simulink model "lab5"  (R2017b)
settings: Solver=VariableStepAuto  StartTime=0.0  StopTime=10.0  RelTol=1e-3
InitFcn:
  | load speech_signal;
  | Fs = 8000;
  | Ts = 1/Fs;
  | 
  | Data_size = 2048;
  | Address_size = 12;
  | Upscale = 32;
undefined symbols (not defined in the file): Radix
libraries: hdlsllib x9, simulink x5, dspmtrx3 x4, dspxfrm3 x2, dspsigops x2, dspvision x1, dspsnks4 x1
settings Model: Creator=Ross_admin  LastModifiedBy=s15z586
settings OptimizationCC: BlockReduction=off  ConditionallyExecuteInputs=off  DefaultParameterBehavior=Inlined
settings DebuggingCC: AlgebraicLoopMsg=error
settings HardwareCC: ProdBitPerPointer=32  ProdBitPerSizeT=32  ProdBitPerPtrDiffT=32  ProdLargestAtomicFloat=None  ProdIntDivRoundTo=Undefined  ProdEndianess=Unspecified  ProdWordSize=32  ProdHWDeviceType=ASIC/FPGA->ASIC/FPGA  TargetBitPerPointer=64  TargetBitPerSizeT=64  TargetBitPerPtrDiffT=64  TargetLongLongMode=on  TargetIntDivRoundTo=Zero  TargetEndianess=LittleEndian  TargetWordSize=64  TargetHWDeviceType=Custom Processor->MATLAB Host Computer  ProdEqTarget=off
settings CodeAppCC: StateflowObjectComments=on

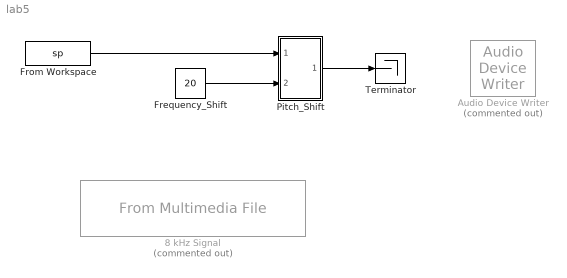
== system lab5 ==
  8 kHz Signal : dspvision/From Multimedia File  Commented=on  inputFilename=SpeechDFT-16-8-mono-5secs.wav  loop=on  numPlays=1  outputStreams=Audio only  videoDataType=single  audioDataType=double  inheritSampleTime=on  userDefinedSampleTime=1/30  noAudioOutput=off  isIntensityVideo=off  fourcc=RGB  colorVideoFormat=Separate color signals  outputEOF=off  dataOrg=Column-major  audioFrameSize=1024  computeAudioFrameSize=off  outSamplingMode=Sample based
      settings: SourceProductBaseCode=VP
  Audio Device Writer : dspsnks4/Audio Device Writer  Commented=on  Driver=DirectSound  Device=Default  InheritSampleRate=on  SampleRate=44100  BitDepth=16-bit integer  BufferSize=4096  NumBuffers=10  DefaultOutputChannelMapping=on  OutputChannelMapping=1:2  OutputNumUnderrunSamples=off  DriverIdx=1  DeviceWarnFlag=''
  Frequency_Shift : Constant  Value=20  OutDataTypeStr=int16
  From Workspace : FromWorkspace  VariableName=sp  SampleTime=Ts
  Pitch_Shift : Subsystem
  Terminator : Terminator
  wires:
  Frequency_Shift/1 -> Pitch_Shift/2(In2)
  From Workspace/1 -> Pitch_Shift/1(In1)
  Pitch_Shift/1(Out1) -> Terminator/1

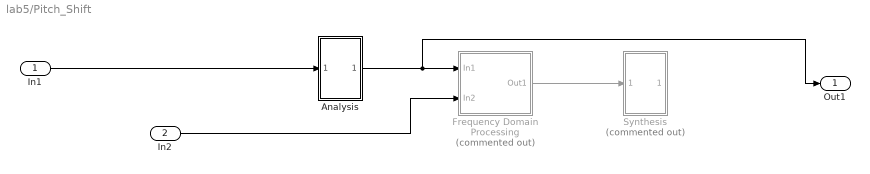
== system lab5/Pitch_Shift ==
  In1 : Inport
  In2 : Inport  Port=2
  Analysis : Subsystem
  Frequency Domain Processing : Subsystem  Commented=on
  Synthesis : Subsystem  Commented=on
  Out1 : Outport
  wires:
  In1/1 -> Analysis/1(In1)
  Frequency Domain Processing/1(Out1) -> Synthesis/1(In1)
  In2/1 -> Frequency Domain Processing/2(In2)
  Analysis/1(Out1) -> Out1/1, Frequency Domain Processing/1(In1)

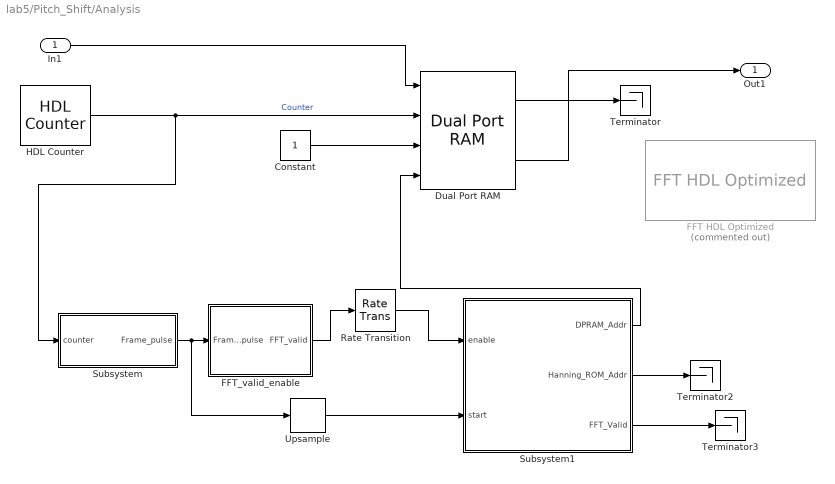
== system lab5/Pitch_Shift/Analysis ==
  In1 : Inport
  Constant : Constant  OutDataTypeStr=boolean  SampleTime=-1
  Dual Port RAM : hdlsllib/HDL RAMs/Dual Port RAM  ram_size=Address_size
      settings: SourceProductName=HDL Coder  SourceProductBaseCode=HD
  FFT HDL Optimized : dspxfrm3/FFT HDL Optimized  Commented=on  FFTLength=1024  Architecture=Burst Radix 2  ComplexMultiplication=Use 3 multipliers and 5 adders  BitReversedOutput=on  BitReversedInput=off  Normalize=off  SimulateUsing=Code generation  RoundingMethod=Floor  ResetInputPort=off  StartOutputPort=off  EndOutputPort=off
      settings: SourceProductName=DSP System Toolbox  SourceProductBaseCode=DS
  FFT_valid_enable : Subsystem
  HDL Counter : hdlsllib/Sources/HDL Counter  CountType=Count limited  CountInit=0  CountStep=1  CountMax=Data_size  CountFromType=Initial value  CountFrom=0  CountResetPort=off  CountLoadPort=off  CountEnbPort=off  CountDirPort=off  CountDataType=Unsigned  CountWordLen=12  CountFracLen=0  CountSampTime=Ts
      settings: SourceProductBaseCode=HD
  Rate Transition : RateTransition  OutPortSampleTime=Ts
  Subsystem : Subsystem
  Subsystem1 : Subsystem
  Terminator : Terminator
  Terminator2 : Terminator
  Terminator3 : Terminator
  Upsample : dspsigops/Upsample  N=4  phase=0  RateOptions=Allow multirate processing  ic=0  mode=Unused parameter value
  Out1 : Outport
  wires:
  In1/1 -> Dual Port RAM/1
  Constant/1 -> Dual Port RAM/3
  HDL Counter/1 -> Subsystem/1("counter "), Dual Port RAM/2  "Counter"
  Subsystem/1(Frame_pulse) -> Upsample/1, FFT_valid_enable/1(Frame_pulse)
  Subsystem1/1(DPRAM_Addr) -> Dual Port RAM/4
  Dual Port RAM/1 -> Terminator/1
  FFT_valid_enable/1(FFT_valid) -> Rate Transition/1
  Subsystem1/2(Hanning_ROM_Addr) -> Terminator2/1
  Subsystem1/3(FFT_Valid) -> Terminator3/1
  Dual Port RAM/2 -> Out1/1
  Rate Transition/1 -> Subsystem1/1(enable)
  Upsample/1 -> Subsystem1/2(start)

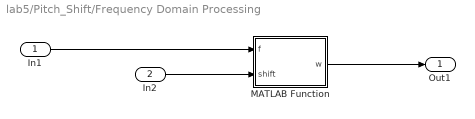
== system lab5/Pitch_Shift/Frequency Domain Processing ==
  In1 : Inport
  In2 : Inport  Port=2
  MATLAB Function : MATLAB Function  TreatAsAtomicUnit=on
  Out1 : Outport
  wires:
  In1/1 -> MATLAB Function/1(f)
  In2/1 -> MATLAB Function/2(shift)
  MATLAB Function/1(w) -> Out1/1

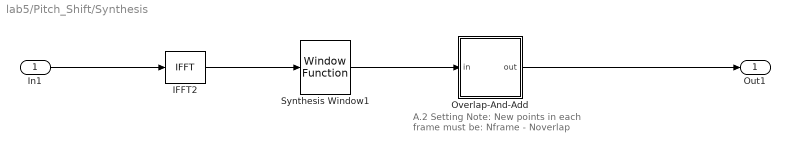
== system lab5/Pitch_Shift/Synthesis ==
  note: A.2
      | Setting Note:
      | New points in each frame must be:
      | Nframe - Noverlap
  In1 : Inport
  IFFT2 : dspxfrm3/IFFT  FFTImplementation=Radix-2  CompMethod=Table lookup  TableOpt=HYBRID  TableOptActive=Speed  BitRevOrder=off  cs_in=on  Normalize=on  InheritFFTLength=on  FFTLength=64  WrapInput=on  mode=Complex  outSamplingMode=Sample based  roundingMode=Floor  overflowMode=off  firstCoeffMode=User-defined  firstCoeffWordLength=16  firstCoeffFracLength=15  firstCoeffDataTypeStr=fixdt(1,16)  firstCoeffLastDataTypeStr=fixdt(1,16)  accumDataTypeStr=Inherit: Same as product output  accumLastDataTypeStr=Inherit: Same as product output  outputMin=[]  outputMax=[]
      settings: SourceProductName=DSP System Toolbox
  Overlap-And-Add : Subsystem  mask(Overlap-And-Add){L=1024 * 1/4}
      mask prompts: L "Number of new points in each frame"
      mask help: Performs overlap-and-add on the input signal. Disjoint frames of the input signal are overlapped with each other for a specified number of points and summed.
      mask Display: disp('Overlap\nAnd\nAdd')
  Synthesis Window1 : dspsigops/Window Function  winmode=Apply window to input  wintype=Hanning  sampmode=Continuous  samptime=1  N=64  Rs=50  beta=10  winsamp=Periodic  UserWindow=hamming  OptParams=off  UserParams={1.0}  dataType=double  isSigned=on  wordLen=16  udDataType=sfix(16)  fracBitsMode=Best precision  numFracBits=15  roundingMode=Floor  overflowMode=off  numSidelobes=4  sidelobeLevel=-30
      settings: SourceProductName=DSP System Toolbox  SourceProductBaseCode=DS
  Out1 : Outport
  wires:
  IFFT2/1 -> Synthesis Window1/1
  Synthesis Window1/1 -> Overlap-And-Add/1(in)
  Overlap-And-Add/1(out) -> Out1/1
  In1/1 -> IFFT2/1

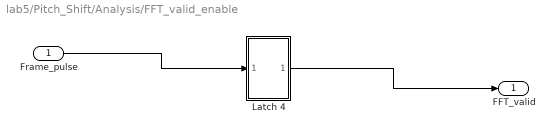
== system lab5/Pitch_Shift/Analysis/FFT_valid_enable ==
  Frame_pulse : Inport
  "Latch 4 " : Subsystem
  FFT_valid : Outport
  wires:
  Frame_pulse/1 -> "Latch 4 "/1(In1)
  "Latch 4 "/1(Out1) -> FFT_valid/1

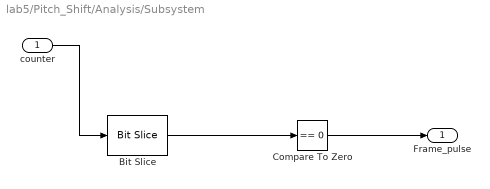
== system lab5/Pitch_Shift/Analysis/Subsystem ==
  "counter " : Inport
  Bit Slice : hdlsllib/Logic and Bit Operations/Bit Slice  lidx=7  ridx=0
  Compare To Zero : simulink/Logic and Bit Operations/Compare To Zero  relop===  OutDataTypeStr=boolean
  Frame_pulse : Outport
  wires:
  "counter "/1 -> Bit Slice/1
  Bit Slice/1 -> Compare To Zero/1
  Compare To Zero/1 -> Frame_pulse/1

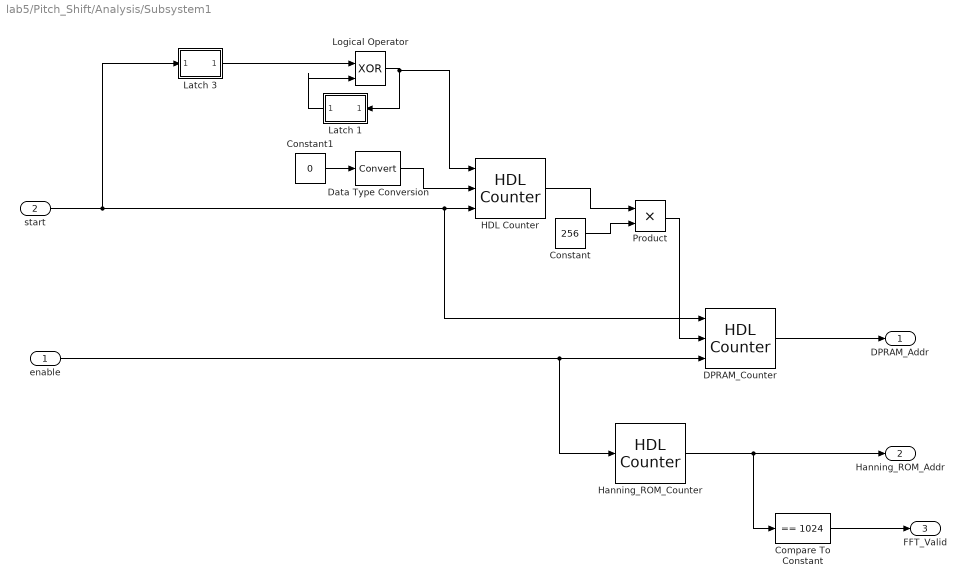
== system lab5/Pitch_Shift/Analysis/Subsystem1 ==
  enable : Inport
  start : Inport  Port=2
  Compare To Constant : simulink/Logic and Bit Operations/Compare To Constant  relop===  const=1024  OutDataTypeStr=boolean
  Constant : Constant  Value=256
  Constant1 : Constant  Value=0
  DPRAM_Counter : hdlsllib/Sources/HDL Counter  CountType=Count limited  CountInit=0  CountStep=1  CountMax=Data_size  CountFromType=Specify  CountFrom=0  CountResetPort=off  CountLoadPort=on  CountEnbPort=on  CountDirPort=off  CountDataType=Unsigned  CountWordLen=12  CountFracLen=0  CountSampTime=1
      settings: SourceProductBaseCode=HD
  Data Type Conversion : DataTypeConversion
  HDL Counter : hdlsllib/Sources/HDL Counter  CountType=Count limited  CountInit=0  CountStep=1  CountMax=1792/256  CountFromType=Initial value  CountFrom=0  CountResetPort=off  CountLoadPort=on  CountEnbPort=on  CountDirPort=off  CountDataType=Unsigned  CountWordLen=Address_size  CountFracLen=0  CountSampTime=1
      settings: SourceProductBaseCode=HD
  "Hanning_ROM_Counter " : hdlsllib/Sources/HDL Counter  CountType=Count limited  CountInit=0  CountStep=1  CountMax=1024  CountFromType=Initial value  CountFrom=0  CountResetPort=off  CountLoadPort=off  CountEnbPort=on  CountDirPort=off  CountDataType=Unsigned  CountWordLen=12  CountFracLen=0  CountSampTime=1
      settings: SourceProductBaseCode=HD
  "Latch 1 " : Subsystem
  Latch 3 : Subsystem
  Logical Operator : Logic  Operator=XOR  IconShape=distinctive  AllPortsSameDT=off  OutDataTypeStr=boolean
  Product : Product  OutDataTypeStr=Inherit: Same as first input
  DPRAM_Addr : Outport
  Hanning_ROM_Addr : Outport  Port=2
  FFT_Valid : Outport  Port=3
  wires:
  DPRAM_Counter/1 -> DPRAM_Addr/1
  "Hanning_ROM_Counter "/1 -> Compare To Constant/1, Hanning_ROM_Addr/1
  enable/1 -> DPRAM_Counter/3, "Hanning_ROM_Counter "/1
  Compare To Constant/1 -> FFT_Valid/1
  start/1 -> Latch 3/1(In1), DPRAM_Counter/1, HDL Counter/3
  HDL Counter/1 -> Product/1
  Product/1 -> DPRAM_Counter/2
  Constant/1 -> Product/2
  Constant1/1 -> Data Type Conversion/1
  Data Type Conversion/1 -> HDL Counter/2
  Logical Operator/1 -> HDL Counter/1, "Latch 1 "/1(In1)
  "Latch 1 "/1(Out1) -> Logical Operator/2
  Latch 3/1(Out1) -> Logical Operator/1

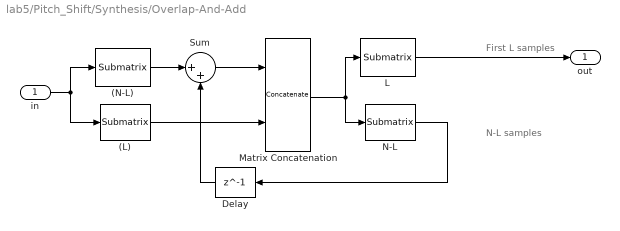
== system lab5/Pitch_Shift/Synthesis/Overlap-And-Add ==
  note: First L samples
  note: N-L samples
  in : Inport
  (L) : dspmtrx3/Submatrix  RowSpan=Range of rows  RowStartMode=Offset from last  RowStartIndex=L-1  RowEndMode=Last  RowEndIndex=1  ColSpan=All columns  ColStartMode=First  ColStartIndex=1  ColEndMode=Last  ColEndIndex=1
  (N-L) : dspmtrx3/Submatrix  RowSpan=Range of rows  RowStartMode=First  RowStartIndex=1  RowEndMode=Offset from last  RowEndIndex=L  ColSpan=All columns  ColStartMode=First  ColStartIndex=1  ColEndMode=Last  ColEndIndex=1
  Delay : Delay  DelayLength=1  InitialCondition=0
  L : dspmtrx3/Submatrix  RowSpan=Range of rows  RowStartMode=First  RowStartIndex=1  RowEndMode=Index  RowEndIndex=L  ColSpan=All columns  ColStartMode=First  ColStartIndex=1  ColEndMode=Last  ColEndIndex=1
  Matrix Concatenation : Concatenate  Mode=Multidimensional array
  N-L : dspmtrx3/Submatrix  RowSpan=Range of rows  RowStartMode=Index  RowStartIndex=L+1  RowEndMode=Last  RowEndIndex=1  ColSpan=All columns  ColStartMode=First  ColStartIndex=1  ColEndMode=Last  ColEndIndex=1
  Sum : Sum  Inputs=|++  SaturateOnIntegerOverflow=on  InputSameDT=on  OutDataTypeStr=Inherit: Same as first input
  out : Outport
  wires:
  L/1 -> out/1
  Sum/1 -> Matrix Concatenation/1
  (N-L)/1 -> Sum/1
  Delay/1 -> Sum/2
  (L)/1 -> Matrix Concatenation/2
  Matrix Concatenation/1 -> L/1, N-L/1
  in/1 -> (L)/1, (N-L)/1
  N-L/1 -> Delay/1

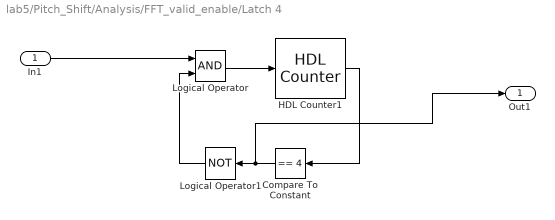
== system lab5/Pitch_Shift/Analysis/FFT_valid_enable/Latch 4  ==
  In1 : Inport
  Compare To Constant : simulink/Logic and Bit Operations/Compare To Constant  relop===  const=4  OutDataTypeStr=boolean
  HDL Counter1 : hdlsllib/Sources/HDL Counter  CountType=Count limited  CountInit=0  CountStep=1  CountMax=4  CountFromType=Initial value  CountFrom=0  CountResetPort=off  CountLoadPort=off  CountEnbPort=on  CountDirPort=off  CountDataType=Unsigned  CountWordLen=3  CountFracLen=0  CountSampTime=1
      settings: SourceProductBaseCode=HD
  Logical Operator : Logic  AllPortsSameDT=off  OutDataTypeStr=boolean
  Logical Operator1 : Logic  Operator=NOT  AllPortsSameDT=off  OutDataTypeStr=boolean
  Out1 : Outport
  wires:
  In1/1 -> Logical Operator/1
  Logical Operator/1 -> HDL Counter1/1
  HDL Counter1/1 -> Compare To Constant/1
  Logical Operator1/1 -> Logical Operator/2
  Compare To Constant/1 -> Out1/1, Logical Operator1/1

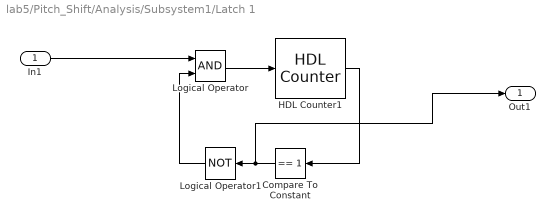
== system lab5/Pitch_Shift/Analysis/Subsystem1/Latch 1  ==
  In1 : Inport
  Compare To Constant : simulink/Logic and Bit Operations/Compare To Constant  relop===  const=1  OutDataTypeStr=boolean
  HDL Counter1 : hdlsllib/Sources/HDL Counter  CountType=Count limited  CountInit=0  CountStep=1  CountMax=4  CountFromType=Initial value  CountFrom=0  CountResetPort=off  CountLoadPort=off  CountEnbPort=on  CountDirPort=off  CountDataType=Unsigned  CountWordLen=3  CountFracLen=0  CountSampTime=1
      settings: SourceProductBaseCode=HD
  Logical Operator : Logic  AllPortsSameDT=off  OutDataTypeStr=boolean
  Logical Operator1 : Logic  Operator=NOT  AllPortsSameDT=off  OutDataTypeStr=boolean
  Out1 : Outport
  wires:
  In1/1 -> Logical Operator/1
  Logical Operator/1 -> HDL Counter1/1
  HDL Counter1/1 -> Compare To Constant/1
  Logical Operator1/1 -> Logical Operator/2
  Compare To Constant/1 -> Out1/1, Logical Operator1/1

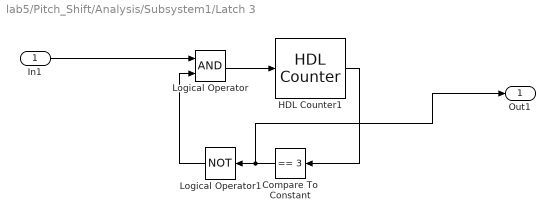
== system lab5/Pitch_Shift/Analysis/Subsystem1/Latch 3 ==
  In1 : Inport
  Compare To Constant : simulink/Logic and Bit Operations/Compare To Constant  relop===  const=3  OutDataTypeStr=boolean
  HDL Counter1 : hdlsllib/Sources/HDL Counter  CountType=Count limited  CountInit=0  CountStep=1  CountMax=4  CountFromType=Initial value  CountFrom=0  CountResetPort=off  CountLoadPort=off  CountEnbPort=on  CountDirPort=off  CountDataType=Unsigned  CountWordLen=3  CountFracLen=0  CountSampTime=1
      settings: SourceProductBaseCode=HD
  Logical Operator : Logic  AllPortsSameDT=off  OutDataTypeStr=boolean
  Logical Operator1 : Logic  Operator=NOT  AllPortsSameDT=off  OutDataTypeStr=boolean
  Out1 : Outport
  wires:
  In1/1 -> Logical Operator/1
  Logical Operator/1 -> HDL Counter1/1
  HDL Counter1/1 -> Compare To Constant/1
  Logical Operator1/1 -> Logical Operator/2
  Compare To Constant/1 -> Out1/1, Logical Operator1/1

== matlab function lab5/Pitch_Shift/Frequency Domain Processing/MATLAB Function ==
  data: f input; w output; shift input
function w = fcn(f,shift)

N = length(f);
w = complex(zeros(N,1));

if shift == 0
    w = f;
else
    
    zf = f(1);            % dc term
    pf = f(2:N/2);        % positive frequencies
    lf = f(N/2 + 1);      % last positive frequency
    nf = f(N/2 + 2:N);  % negative frequencies (paired with positive frequencies)
    
    w(1) = zf;
    w(N/2+1) = complex(0);                   % just zero frequency at -pi since both positive and negative frequencies map here when shifted
        
    if shift > 0  % increase the frequencies
        
        for i=1:shift
            w(i) = complex(0);                   % fill in vacated positive frequencies with zeros
        end
        w(shift+1:N/2) = pf(1:end-shift+1);      % shift positive frequencies to the right

        w(N/2+2:end-shift) = nf(shift + 1:end);  % shift negative frequencies to the left
        for i=N-shift+1:N
            w(i) = complex(0);                   % fill in vacated negative frequencies with zeros
        end
        
    end
    if shift < 0  % decrease the frequencies
      
        nshift = abs(shift);
        
        w(2:N/2-nshift) = pf(nshift+1:end);      % shift positive frequencies to the left
        for i=N/2-nshift+2:N/2+1
            w(i) = complex(0);                   % fill in vacated positive frequencies with zeros
        end
        
        w(N/2+2+nshift:N) = nf(1:end-nshift);      % shift negative frequencies to the right
        for i=N/2+2:N/2+2+nshift-1
            w(i) = complex(0);                   % fill in vacated negative frequencies with zeros
        end
        


    end
end
